simulink model "TEST_LIDAR"  (R2022b)
settings: Solver=FixedStepAuto  StartTime=0.0  StopTime=inf  FixedStep=1e-3  RelTol=1e-3  EnableMultiTasking=on
model workspace (MAT data in the model file):
  SL_ROS_VariableLengthArrays_MaxSizes : object (value not decoded)
values from neighbouring files (symbols this model uses):
  data = theClient.GetLastFrameOfData()    [FuncMotive.m]
undefined symbols (not defined in the file or in its folder): angular, carstamp, CIRCUIT, CLTF_DAMP, CLTF_FREQ, CLTF_GAIN, CONTROL, CONTROL_INI, DiscIntNeverNeededParam, INPUT, linear, MCP3201, MD25, MODEL, MODEL_INI, mpcstate, MPU60X0, MPU9250, MSG, NAV_MPC_CONTROL, OUTPUT, RCRX, SAMPLING_TIME, SYSID_INPUT, VL6180X
libraries: raspberrypiCommlib x160, simulink x89, raspberrypiNetworklib x22, ros2lib x14, dspsigattribs x14, embedlinuxBasiclib x12, ctrlSharedLib x2, mpclib x1, vrlib x1, sldrtlib x1
(part 13 of 19)

== matlab function TEST_LIDAR/CONTROL/STATE MACHINE UPDATE ==
  data: CONTROL_IN input Bus: CONTROL_Bus; CONTROL output Bus: CONTROL_Bus; MSG_IN input; MSG output Bus: MSG_Bus
function [CONTROL,MSG] = STATE_MACHINE(CONTROL_IN,MSG_IN)

%--------------------------------------------------------------
% COPY BUSES
%--------------------------------------------------------------
CONTROL = CONTROL_IN; 
MSG = MSG_IN;

%--------------------------------------------------------------
% TIMING
%--------------------------------------------------------------
% SAMPLING TIME
SAMPLING_TIME = CONTROL.PARAM.SAMPLING_TIME; % s
% 6-bit SAMPLING COUNTER
SAMPLING_COUNT = CONTROL.STATE.SAMPLING_COUNT;
SAMPLING_COUNT = SAMPLING_COUNT + uint8(1);
if SAMPLING_COUNT > uint8(63) 
    SAMPLING_COUNT = uint8(0);
end
CONTROL.STATE.SAMPLING_COUNT = SAMPLING_COUNT;
% TIMER
TIMER = CONTROL.STATE.TIMER;
% DELAY IN CONTROL ACTIVATION
CONTROL_ACT_DELAY = CONTROL.PARAM.CONTROL_ACT_DELAY;

%--------------------------------------------------------------
% SYSTEM OPERATION STATUS
%--------------------------------------------------------------
% / 0. BOOTING     / 1. SENSOR CALIBRATION / 2.  READY
% / 3. OPEN LOOP   / 4. ATTITUDE           / 5.  VELOCITY  
% / 6. NAVIGATION  / 7. WALL FOLLOWER      / 8.  NAVIGATION COMPETITION 
% / 9. WALL FOLLOWER COMPETITION           /10.  FORWARD VELOCITY COMPETITION
% /11. STOP        / 12. SELF-BALANCE      /13.  SBV CALIBRATION 
CURRENT_STATUS_SYS = CONTROL.STATE.CURRENT_STATUS_SYS;
NEXT_STATUS = CURRENT_STATUS_SYS;

%--------------------------------------------------------------
% PC OPERATION STATUS
%--------------------------------------------------------------
% / 0. CONTROL CONFIGURATION   / 1. WAITING FOR RPI SET UP  /
% / 2. MONITORIZATION / 3. STOP /
CURRENT_STATUS_PC = CONTROL.STATE.CURRENT_STATUS_PC;

%--------------------------------------------------------------
% CONTROL MODE
%--------------------------------------------------------------
% / 0. OPEN LOOP / 1. FORWARD VELOCITY AND YAW ANGLE / 
% / 2. FORWARD VELOCITY AND YAW RATE / 3. NAVIGATION / 
% / 4. WALL FOLLOWER / 5. WALL FOLLOWING COMPETITION /
% / 6. NAVIGATION COMPETITION / 7. FORWARD VELOCITY COMPETITION /
% / 8. SELF-BALANCE 
CONTROL_MODE = CONTROL.STATE.CONTROL_MODE;

%--------------------------------------------------------------
% CONTROL STATUS
%--------------------------------------------------------------
% / 0. INITIALIZATION  / 1. ESTIMATION  / 2. ACTIVE CONTROL
CONTROL_STATUS = CONTROL.STATE.CONTROL_STATUS;

%--------------------------------------------------------------
% MOTOR MODE
%--------------------------------------------------------------
% / 0. NOT ENABLED / 1. ENABLED 
MOTOR_MODE = CONTROL.STATE.MOTOR_MODE;

%--------------------------------------------------------------
% COMMUNICATIONS
%--------------------------------------------------------------
% COMMUNICATIONS MODE
% / 0. NOT ENABLED / 1. ENABLED / 2. BLACKBOX
COMM_MODE = CONTROL.STATE.COMM_MODE;
% UART MODE
% / 0. NOT ENABLED / 1. ENABLED
UART_MODE = CONTROL.STATE.UART_MODE;

%--------------------------------------------------------------
% INPUTS
%--------------------------------------------------------------
BUTTONS = CONTROL.STATE.BUTTONS;

%--------------------------------------------------------------
% PERSISTENT VARIABLES
%--------------------------------------------------------------
persistent initialize ACC_ERR MCS_EARTH_POS_OFFS MCS_EULER_ANG_OFFS ...
           NAV_EARTH_POS_OFFS NAV_EULER_ANG_OFFS IMU_PITCH_ANG_INI ...
           NUM_MSRT_LIDAR_2D TIMER_NAV
if isempty(initialize)
    ACC_ERR = 0;
    MCS_EARTH_POS_OFFS = zeros(3,1);
    MCS_EULER_ANG_OFFS = zeros(3,1);
    NAV_EARTH_POS_OFFS = zeros(3,1);
    NAV_EULER_ANG_OFFS = zeros(3,1);   
    IMU_PITCH_ANG_INI = 0;
    NUM_MSRT_LIDAR_2D = zeros(360,1);
    TIMER_NAV = 0;
    initialize = 1;
end

%--------------------------------------------------------------
% STATUS UPDATE
%--------------------------------------------------------------
switch CURRENT_STATUS_SYS
    
    %----------------------------------------------------------------------
    case 0 % BOOTING
    %----------------------------------------------------------------------
        % CONTROL STATUS: INITIALIZATION
        CONTROL_STATUS = uint8(0);     
        % MOTOR MODE: SHUTDOWN
        MOTOR_MODE = uint8(0);
        % LIDAR 2D
        if CONTROL.STATE.WALL_FOLLOWER_MODE
            CONTROL.STATE.LIDAR_2D_MODE = uint8(0);
        end
        % LEDs
        CONTROL.OUTPUT.LEDS = uint8([0 0 0]');
        % COMPETITION LIMITATION
        CONTROL.STATE.MAX_FORWARD_VEL_REACHED = uint8(0);
        % COMPETITION TIME AND ACCUMULATED ERROR
        CONTROL.STATE.COMP_TIME = 0;
        ACC_ERR = 0;
        % COMMUNICATIONS
        if COMM_MODE > 0
            BUFFER_RX = MSG.RX_BUFFER;
            NUM_MSG_RX = BUFFER_RX(1);
            if NUM_MSG_RX>0
                HEADER_RX = BUFFER_RX(1:2*NUM_MSG_RX+1);
                ID_RX = HEADER_RX(2:2:end);
                MSG.TX_ID = zeros(8,1,'uint8');
                if UART_MODE == 1
                    MSG.TX_ID(1:length(ID_RX)) = ID_RX(1:end)';
                else
                    MSG.TX_ID(1:length(ID_RX)) = [uint8(1) ID_RX(2:end)']';
                end
                if (BUTTONS(1) && (CURRENT_STATUS_PC == 1)) % BUTTON A
                    NEXT_STATUS = uint8(1); % SENSOR CALIBRATION
                    % TIMER RESET
                    TIMER = 0;
                end
            end
        else
            if BUTTONS(1) % BUTTON A
                NEXT_STATUS = uint8(1); % SENSOR CALIBRATION
                % TIMER RESET
                TIMER = 0;
            end
        end

    %----------------------------------------------------------------------
    case 1 % SENSOR CALIBRATION
    %----------------------------------------------------------------------
         % LIDAR 2D
        if CONTROL.STATE.WALL_FOLLOWER_MODE
            CONTROL.STATE.LIDAR_2D_MODE = uint8(1);
        end
        if TIMER >= 10
            if CONTROL.STATE.VEHICLE_MODE == 1 
                CONTROL.OUTPUT.LEDS = uint8([1 1 0]');
                if BUTTONS(1) % BUTTON A
                    NEXT_STATUS = uint8(13); % SVF CALIBRATION
                    % TIMER RESET
                    TIMER = 0;
                else
                    NEXT_STATUS = uint8(1); % SENSOR CALIBRATION
                end
            else
                NEXT_STATUS = uint8(2); % READY
            end
            % MOTION CAPTURE SYSTEM OFFSET
            CONTROL.PARAM.MCS_EARTH_POS_OFFS = MCS_EARTH_POS_OFFS;  
            CONTROL.PARAM.MCS_EULER_ANG_OFFS = MCS_EULER_ANG_OFFS; 
            % NAVIGATION SYSTEM OFFSET
            CONTROL.PARAM.NAV_EARTH_POS_OFFS = NAV_EARTH_POS_OFFS;
            CONTROL.PARAM.NAV_EULER_ANG_OFFS = NAV_EULER_ANG_OFFS;
        else
            % UPDATE TIMER
            TIMER = TIMER + SAMPLING_TIME;
            % LEDs
            CONTROL.OUTPUT.LEDS = uint8([0 0 1]');
            % MOTION CAPTURE SYSTEM CALIBRATION
            if CONTROL.STATE.MCS_MODE==1 || CONTROL.STATE.NAV_MODE==1
                ALFA_CALIB = CONTROL.PARAM.MCS_ALFA_CALIB;
                MCS_EARTH_POS_OFFS = ALFA_CALIB*MCS_EARTH_POS_OFFS + ...
                    (1-ALFA_CALIB)*CONTROL.INPUT.MCS_EARTH_POS;
                MCS_EULER_ANG_OFFS = ALFA_CALIB*MCS_EULER_ANG_OFFS + ...
                    (1-ALFA_CALIB)*CONTROL.INPUT.MCS_EULER_ANG;
            end            
            if CONTROL.STATE.NAV_MODE==3
                ALFA_CALIB = CONTROL.PARAM.NAV_ALFA_CALIB;
                NAV_EARTH_POS_OFFS = ALFA_CALIB*NAV_EARTH_POS_OFFS + ...
                    (1-ALFA_CALIB)*CONTROL.INPUT.NAV_EARTH_POS;
                NAV_EULER_ANG_OFFS = ALFA_CALIB*NAV_EULER_ANG_OFFS + ...
                    (1-ALFA_CALIB)*CONTROL.INPUT.NAV_EULER_ANG;
            end  
            if CONTROL.STATE.NAV_MODE==2
                for nn = 1:size(CONTROL.INPUT.LIDAR_2D,1)
                    if CONTROL.INPUT.LIDAR_2D(nn,2)>0
                        CONTROL.PARAM.LIDAR_2D_MAP(nn) = ...
                            (CONTROL.PARAM.LIDAR_2D_MAP(nn)*NUM_MSRT_LIDAR_2D(nn) + ...
                            CONTROL.INPUT.LIDAR_2D(nn,2))/(NUM_MSRT_LIDAR_2D(nn)+1);
                        NUM_MSRT_LIDAR_2D(nn) = NUM_MSRT_LIDAR_2D(nn) + 1;
                   end
                end
            end
        end
        % CONTROL STATUS: INITIALIZATION
        CONTROL_STATUS = uint8(0);     
        % MOTOR MODE: NOT ENABLED
        MOTOR_MODE = uint8(0); 
        % COMMUNICATIONS
        if (COMM_MODE >= 1) && (UART_MODE == 1)
            MSG.TX_ID = uint8([139 140 141 142 143 144 0 0]');
        elseif (COMM_MODE >= 1) && (UART_MODE == 0)
            MSG.TX_ID = uint8([1 139 140 141 142 143 144 0]');
        else
            MSG.TX_ID = uint8([0 0 0 0 0 0 0 0]');
        end

    %----------------------------------------------------------------------
    case 2 % READY
    %----------------------------------------------------------------------
        if BUTTONS(1) % BUTTON A
            if CONTROL_MODE == 0 % OPEN LOOP
                NEXT_STATUS = uint8(3); 
            elseif CONTROL_MODE == 1 % FORWARD VELOCITY AND YAW ANGLE
                NEXT_STATUS = uint8(4); 
            elseif CONTROL_MODE == 2 % FORWARD VELOCITY AND YAW RATE
                NEXT_STATUS = uint8(5); 
            elseif CONTROL_MODE == 3 % NAVIGATION
                NEXT_STATUS = uint8(6); 
            elseif CONTROL_MODE == 4 % WALL FOLLOWER
                NEXT_STATUS = uint8(7); 
            elseif CONTROL_MODE == 5 % WALL-FOLLOWER COMPETITION
                NEXT_STATUS = uint8(8); 
            elseif CONTROL_MODE == 6 % NAVIGATION COMPETITION
                NEXT_STATUS = uint8(9); 
            elseif CONTROL_MODE == 7 % FORWARD VELOCITY COMPETITION
                NEXT_STATUS = uint8(10);   
            elseif CONTROL_MODE == 8 % SELF-BALANCE
                NEXT_STATUS = uint8(12); 
            else
                NEXT_STATUS = uint8(11);
            end            
        end  
        % CONTROL STATUS: INITIALIZATION
        CONTROL_STATUS = uint8(0);              
        % MOTOR MODE: NOT ENABLED
        MOTOR_MODE = uint8(0); 
        % EKF MODE: NOT ENABLED
        CONTROL.EKF_IMU.ESTIMATION_MODE = uint8(0);
        CONTROL.EKF_WFL.ESTIMATION_MODE = uint8(0);
        % LEDs
        CONTROL.OUTPUT.LEDS = uint8([0 1 0]');
        % TARGETS
        CONTROL.TARGET.MOTOR_VOLT_CD_REF = zeros(2,1);
        CONTROL.TARGET.YAW_ANG_REF = 0;
        CONTROL.TARGET.FORWARD_VEL_REF = 0;
        CONTROL.TARGET.YAW_RATE_REF = 0;
        CONTROL.TARGET.WALL_DIST_REF = 0;
        % COMMUNICATIONS            
        if (COMM_MODE >= 1) && (UART_MODE == 1)
            MSG.TX_ID = uint8([139 140 141 142 143 144 0 0]');
        elseif (COMM_MODE >= 1) && (UART_MODE == 0)
            MSG.TX_ID = uint8([1 139 140 141 142 143 144 0]');
        else
            MSG.TX_ID = uint8([0 0 0 0 0 0 0 0]');
        end
        
    %----------------------------------------------------------------------
    case 3 % OPEN LOOP
    %----------------------------------------------------------------------
        if TIMER >= CONTROL_ACT_DELAY % Delay in control activation
            NEXT_STATUS = uint8(3);
            % CONTROL STATUS: ACTIVE CONTROL
            CONTROL_STATUS = uint8(2);
            % MOTOR MODE: ENABLED
            MOTOR_MODE = uint8(1);                       
           % LEDs
            CONTROL.OUTPUT.LEDS = uint8([0 0 0]');
            % TARGETS
            CONTROL.TARGET.MOTOR_VOLT_CD_REF = ...
                CONTROL.TARGET.MOTOR_VOLT_CD_REF_LC.*(CONTROL.STATE.MV_TARGET_SOURCE==0) + ...
                CONTROL.TARGET.MOTOR_VOLT_CD_REF_PC.*(CONTROL.STATE.MV_TARGET_SOURCE==1) + ...
                CONTROL.TARGET.MOTOR_VOLT_CD_REF_RC.*(CONTROL.STATE.MV_TARGET_SOURCE>=2);
            % BUTTON B
            if BUTTONS(2) == 1
                NEXT_STATUS = uint8(11); % STOP
                % TIMER_1 RESET
                TIMER = 0;                
            end
        else
            % UPDATE TIMER
            TIMER = TIMER + SAMPLING_TIME;
            % CONTROL STATUS: INITIALIZATION
            CONTROL_STATUS = uint8(0);
            % MOTOR MODE: NOT ENABLED
            MOTOR_MODE = uint8(0);
        end
        % COMMUNICATIONS
        if (COMM_MODE >= 1) && (UART_MODE == 1)
            MSG.TX_ID = uint8([139 140 141 142 143 144 0 0]');
        elseif (COMM_MODE >= 1) && (UART_MODE == 0)
            MSG.TX_ID = uint8([1 139 140 141 142 143 144 0]');
        else
            MSG.TX_ID = uint8([0 0 0 0 0 0 0 0]');
        end

    %----------------------------------------------------------------------
    case 4 % FORWARD VELOCITY AND YAW ANGLE
    %----------------------------------------------------------------------
        if TIMER >= CONTROL_ACT_DELAY % Delay in control activation
            NEXT_STATUS = uint8(4);
            % CONTROL STATUS: ACTIVE CONTROL
            CONTROL_STATUS = uint8(2);
            % MOTOR MODE: ENABLED
            MOTOR_MODE = uint8(1);                      
            % LEDs
            CONTROL.OUTPUT.LEDS = uint8([0 0 0]');
            % TARGETS
            CONTROL.TARGET.FORWARD_VEL_REF = ...
                CONTROL.TARGET.FORWARD_VEL_REF_LC.*(CONTROL.STATE.FV_TARGET_SOURCE==0) + ...
                CONTROL.TARGET.FORWARD_VEL_REF_PC.*(CONTROL.STATE.FV_TARGET_SOURCE==1) + ...
                CONTROL.TARGET.FORWARD_VEL_REF_RC.*(CONTROL.STATE.FV_TARGET_SOURCE>=2);
            CONTROL.TARGET.YAW_ANG_REF = ...
                CONTROL.TARGET.YAW_ANG_REF_LC.*(CONTROL.STATE.YA_TARGET_SOURCE==0) + ...
                CONTROL.TARGET.YAW_ANG_REF_PC.*(CONTROL.STATE.YA_TARGET_SOURCE==1) + ...
                CONTROL.TARGET.YAW_ANG_REF_RC.*(CONTROL.STATE.YA_TARGET_SOURCE>=2);
            % BUTTON B
            if BUTTONS(2) == 1
                NEXT_STATUS = uint8(11); % STOP
                % TIMER RESET
                TIMER = 0;                
            end
        else      
            % UPDATE TIMER
            TIMER = TIMER + SAMPLING_TIME;
            % CONTROL STATUS: INITIALIZATION
            CONTROL_STATUS = uint8(0);
            % MOTOR MODE: NOT ENABLED
            MOTOR_MODE = uint8(0);
        end
        % COMMUNICATIONS
        if (COMM_MODE >= 1) && (UART_MODE == 1)
            MSG.TX_ID = uint8([139 140 141 142 143 144 0 0]');
        elseif (COMM_MODE >= 1) && (UART_MODE == 0)
            MSG.TX_ID = uint8([1 139 140 141 142 143 144 0]');
        else
            MSG.TX_ID = uint8([0 0 0 0 0 0 0 0]');
        end

    %----------------------------------------------------------------------
    case 5 % FORWARD VELOCITY AND YAW RATE
    %----------------------------------------------------------------------
        if TIMER >= CONTROL_ACT_DELAY % Delay in control activation
            NEXT_STATUS = uint8(5);
            % CONTROL STATUS: ACTIVE CONTROL
            CONTROL_STATUS = uint8(2);
            % MOTOR MODE: ENABLED
            MOTOR_MODE = uint8(1);            
            % LEDs
            CONTROL.OUTPUT.LEDS = uint8([0 0 0]');
            % TARGETS
            CONTROL.TARGET.FORWARD_VEL_REF = ...
                CONTROL.TARGET.FORWARD_VEL_REF_LC.*(CONTROL.STATE.FV_TARGET_SOURCE==0) + ...
                CONTROL.TARGET.FORWARD_VEL_REF_PC.*(CONTROL.STATE.FV_TARGET_SOURCE==1) + ...
                CONTROL.TARGET.FORWARD_VEL_REF_RC.*(CONTROL.STATE.FV_TARGET_SOURCE>=2);
            CONTROL.TARGET.YAW_RATE_REF = ...
                CONTROL.TARGET.YAW_RATE_REF_LC.*(CONTROL.STATE.YR_TARGET_SOURCE==0) + ...
                CONTROL.TARGET.YAW_RATE_REF_PC.*(CONTROL.STATE.YR_TARGET_SOURCE==1) + ...
                CONTROL.TARGET.YAW_RATE_REF_RC.*(CONTROL.STATE.YR_TARGET_SOURCE>=2);
            % BUTTON B
            if BUTTONS(2) == 1
                NEXT_STATUS = uint8(11); % STOP
                % TIMER RESET
                TIMER = 0;                
            end
        else      
            % UPDATE TIMER
            TIMER = TIMER + SAMPLING_TIME;
            % CONTROL STATUS: INITIALIZATION
            CONTROL_STATUS = uint8(0);
            % MOTOR MODE: NOT ENABLED
            MOTOR_MODE = uint8(0);
        end
         % COMMUNICATIONS
        if (COMM_MODE >= 1) && (UART_MODE == 1)
            MSG.TX_ID = uint8([139 140 141 142 143 144 0 0]');
        elseif (COMM_MODE >= 1) && (UART_MODE == 0)
            MSG.TX_ID = uint8([1 139 140 141 142 143 144 0]');
        else
            MSG.TX_ID = uint8([0 0 0 0 0 0 0 0]');
        end

    %----------------------------------------------------------------------
    case 6 % NAVIGATION
    %----------------------------------------------------------------------
        if TIMER >= CONTROL_ACT_DELAY % Delay in control activation
            NEXT_STATUS = uint8(6);
            % CONTROL STATUS: ACTIVE CONTROL
            CONTROL_STATUS = uint8(2);
            % MOTOR MODE: ENABLED
            MOTOR_MODE = uint8(1);
            % BUTTON B
            if BUTTONS(2) == 1
                NEXT_STATUS = uint8(11); % STOP
                % TIMER RESET
                TIMER = 0;                
            end
            % LEDs
            CONTROL.OUTPUT.LEDS = uint8([0 0 0]');
            % TARGETS
            if CONTROL.STATE.NAV_TARGET_SOURCE==0 % LOCAL
                CONTROL.TARGET.NAV_REF = CONTROL.TARGET.NAV_REF_LC;
            elseif CONTROL.STATE.NAV_TARGET_SOURCE==1 % PC
                CONTROL.TARGET.NAV_REF = CONTROL.TARGET.NAV_REF_PC;
            elseif CONTROL.STATE.NAV_TARGET_SOURCE==2 || CONTROL.STATE.NAV_TARGET_SOURCE==3 % RC
                CONTROL.TARGET.NAV_REF = CONTROL.TARGET.NAV_REF_RC;
            elseif CONTROL.STATE.NAV_TARGET_SOURCE==4 % MISSION
                % Number of waypoints
                NUM_WAYPOINTS = CONTROL.PARAM.MISSION_NUM_WAYPOINTS;
                % Waypoint list
                WP_LIST = CONTROL.PARAM.MISSION_WAYPOINTS(1:NUM_WAYPOINTS,:);
                % Next waypoint
                NEXT_WP = CONTROL.PARAM.MISSION_COUNT;
                % Tolerances
                WP_RADIUS = CONTROL.PARAM.MISSION_WP_RADIUS;
                % References
                CONTROL.TARGET.NAV_REF = WP_LIST(NEXT_WP,2:3)';
                % POSITION UPDATE
                % Current position and yaw angle
                NAV_MO = CONTROL.INPUT.NAV_MO;
                % Check waypoint
                POS_DIST = sqrt(sum((CONTROL.TARGET.NAV_REF - NAV_MO).^2));
                % Increase waypoint
                if POS_DIST<WP_RADIUS
                    if WP_LIST(NEXT_WP,1)>TIMER_NAV
                        TIMER_NAV = TIMER_NAV + SAMPLING_TIME;
                    else
                        TIMER_NAV = 0;
                        NEXT_WP = NEXT_WP + uint8(1);
                    end
                end
                if NEXT_WP>size(WP_LIST,1)
                    NEXT_WP = uint8(size(WP_LIST,1));
                end
                % CONTROL BUS UPDATE FOR COMPETITION
                CONTROL.PARAM.MISSION_COUNT = NEXT_WP;
            else
                % NEXT STATUS: READY
                NEXT_STATUS = uint8(2);
                % MOTOR MODE: SHUT DOWN
                MOTOR_MODE = uint8(0);
            end
            CONTROL.TARGET.POS_XY_REF = CONTROL.TARGET.NAV_REF;
            % BUTTON B
            if BUTTONS(2) == 1
                NEXT_STATUS = uint8(11); % STOP
                % TIMER RESET
                TIMER = 0;
            end
        else
            % UPDATE TIMER
            TIMER = TIMER + SAMPLING_TIME;
            % CONTROL STATUS: INITIALIZATION
            CONTROL_STATUS = uint8(0);
            % MOTOR MODE: NOT ENABLED
            MOTOR_MODE = uint8(0);
        end
        % COMMUNICATIONS
        if (COMM_MODE >= 1) && (UART_MODE == 1)
            MSG.TX_ID = uint8([139 140 141 142 143 144 0 0]');
        elseif (COMM_MODE >= 1) && (UART_MODE == 0)
            MSG.TX_ID = uint8([1 139 140 141 142 143 144 0]');
        else
            MSG.TX_ID = uint8([0 0 0 0 0 0 0 0]');
        end
        
    %----------------------------------------------------------------------
    case 7 % WALL FOLLOWER
    %----------------------------------------------------------------------
        if TIMER >= CONTROL_ACT_DELAY % Delay in control activation
            NEXT_STATUS = uint8(7);
            % CONTROL STATUS: ACTIVE CONTROL
            CONTROL_STATUS = uint8(2);
            % MOTOR MODE: ENABLED
            MOTOR_MODE = uint8(1); 
            % LIDAR 2D
            if CONTROL.STATE.WALL_FOLLOWER_MODE
                CONTROL.STATE.LIDAR_2D_MODE = uint8(1);
            end
            % LEDs
            CONTROL.OUTPUT.LEDS = uint8([0 0 0]');
            % TARGETS
            CONTROL.TARGET.FORWARD_VEL_REF = ...
                CONTROL.TARGET.FORWARD_VEL_REF_LC.*(CONTROL.STATE.FV_TARGET_SOURCE==0) + ...
                CONTROL.TARGET.FORWARD_VEL_REF_PC.*(CONTROL.STATE.FV_TARGET_SOURCE==1) + ...
                CONTROL.TARGET.FORWARD_VEL_REF_RC.*(CONTROL.STATE.FV_TARGET_SOURCE>=2);
            CONTROL.TARGET.WALL_DIST_REF = ...
                CONTROL.TARGET.WALL_DIST_REF_LC.*(CONTROL.STATE.WD_TARGET_SOURCE==0) + ...
                CONTROL.TARGET.WALL_DIST_REF_PC.*(CONTROL.STATE.WD_TARGET_SOURCE==1) + ...
                CONTROL.TARGET.WALL_DIST_REF_RC.*(CONTROL.STATE.WD_TARGET_SOURCE>=2);
            % BUTTON B
            if BUTTONS(2) == 1
                NEXT_STATUS = uint8(11); % STOP
                % TIMER RESET
                TIMER = 0;                
            end
        else      
            % UPDATE TIMER
            TIMER = TIMER + SAMPLING_TIME;
            % CONTROL STATUS: INITIALIZATION
            CONTROL_STATUS = uint8(0);
            % MOTOR MODE: NOT ENABLED
            MOTOR_MODE = uint8(0);
        end        
        % COMMUNICATIONS
        if (COMM_MODE >= 1) && (UART_MODE == 1)
            MSG.TX_ID = uint8([139 140 141 142 143 144 0 0]');
        elseif (COMM_MODE >= 1) && (UART_MODE == 0)
            MSG.TX_ID = uint8([1 139 140 141 142 143 144 0]');
        else
            MSG.TX_ID = uint8([0 0 0 0 0 0 0 0]');
        end

    %----------------------------------------------------------------------
    case 8 % WALL-FOLLOWER COMPETITION
    %----------------------------------------------------------------------
        if TIMER >= CONTROL_ACT_DELAY % Delay in control activation
            NEXT_STATUS = uint8(8);
            % CONTROL STATUS: ACTIVE CONTROL
            CONTROL_STATUS = uint8(2);
            % MOTOR MODE: ENABLED
            MOTOR_MODE = uint8(1);
            % LIDAR 2D
            if CONTROL.STATE.WALL_FOLLOWER_MODE
                CONTROL.STATE.LIDAR_2D_MODE = uint8(1);
            end            % LEDs
            CONTROL.OUTPUT.LEDS = uint8([0 0 0]');
            % TARGETS
            CONTROL.TARGET.FORWARD_VEL_REF = ...
                CONTROL.TARGET.FORWARD_VEL_REF_LC.*(CONTROL.STATE.FV_TARGET_SOURCE==0) + ...
                CONTROL.TARGET.FORWARD_VEL_REF_PC.*(CONTROL.STATE.FV_TARGET_SOURCE==1) + ...
                CONTROL.TARGET.FORWARD_VEL_REF_RC.*(CONTROL.STATE.FV_TARGET_SOURCE>=2);
            CONTROL.TARGET.WALL_DIST_REF = ...
                CONTROL.TARGET.WALL_DIST_REF_LC.*(CONTROL.STATE.WD_TARGET_SOURCE==0) + ...
                CONTROL.TARGET.WALL_DIST_REF_PC.*(CONTROL.STATE.WD_TARGET_SOURCE==1) + ...
                CONTROL.TARGET.WALL_DIST_REF_RC.*(CONTROL.STATE.WD_TARGET_SOURCE>=2);       
            % FORWARD VELOCITY LIMITATION
            if CONTROL.INPUT.FORWARD_VEL>0.5
                CONTROL.STATE.MAX_FORWARD_VEL_REACHED = uint8(1);
            end
            if CONTROL.STATE.MAX_FORWARD_VEL_REACHED
                CONTROL.TARGET.FORWARD_VEL_REF = 0;
            end
            % BUTTON B
            if BUTTONS(2) == 1
                NEXT_STATUS = uint8(11); % STOP
                % TIMER RESET
                TIMER = 0;                
            end
        else      
            % UPDATE TIMER
            TIMER = TIMER + SAMPLING_TIME;
            % CONTROL STATUS: INITIALIZATION
            CONTROL_STATUS = uint8(0);
            % MOTOR MODE: NOT ENABLED
            MOTOR_MODE = uint8(0);
        end
        % COMMUNICATIONS
        if (COMM_MODE >= 1) && (UART_MODE == 1)
            MSG.TX_ID = uint8([139 140 141 142 143 144 0 0]');
        elseif (COMM_MODE >= 1) && (UART_MODE == 0)
            MSG.TX_ID = uint8([1 139 140 141 142 143 144 0]');
        else
            MSG.TX_ID = uint8([0 0 0 0 0 0 0 0]');
        end

    %----------------------------------------------------------------------
    case 9 % NAVIGATION COMPETITION
    %----------------------------------------------------------------------
        if TIMER >= CONTROL_ACT_DELAY % Delay in control activation
            NEXT_STATUS = uint8(9);
            % CONTROL STATUS: ACTIVE CONTROL
            CONTROL_STATUS = uint8(2);
            % MOTOR MODE: ENABLED
            MOTOR_MODE = uint8(1);
            % BUTTON B
            if BUTTONS(2) == 1
                NEXT_STATUS = uint8(11); % STOP
                % TIMER RESET
                TIMER = 0;                
            end
            % LEDs
            CONTROL.OUTPUT.LEDS = uint8([0 0 0]');
            % POSITION UPDATE
            WP_XY = CONTROL.PARAM.MISSION_WAYPOINTS(1:CONTROL.PARAM.MISSION_NUM_WAYPOINTS,2:3)';
            WP_R = CONTROL.PARAM.MISSION_WP_RADIUS;
            NAV_MO = CONTROL.INPUT.NAV_MO;
            NEXT_WP = CONTROL.PARAM.MISSION_COUNT;
            POS_INC = (WP_XY(1,NEXT_WP) - NAV_MO(1)) + (WP_XY(2,NEXT_WP) - NAV_MO(2))*1i;
            POS_INC_MAG = abs(POS_INC);
            % COMPETITION TIME UPDATE
            COMP_START_TIME = CONTROL.STATE.COMP_START_TIME;
            COMP_TIME = CONTROL.STATE.COMP_TIME;
            if COMP_START_TIME>0 && POS_INC_MAG<WP_R && NEXT_WP==1
                CONTROL.STATE.COMP_STARTED = uint8(1);
            end
            if CONTROL.STATE.COMP_STARTED && CONTROL.STATE.COMP_FINISHED==0
                COMP_TIME = COMP_TIME + SAMPLING_TIME;
            else
                COMP_START_TIME = COMP_START_TIME + SAMPLING_TIME*(CONTROL.STATE.COMP_STARTED==0);
            end
            if POS_INC_MAG<WP_R && CONTROL.STATE.COMP_STARTED
                 NEXT_WP = NEXT_WP + uint8(1);
            end
            if NEXT_WP>size(WP_XY,2)
                NEXT_WP = uint8(size(WP_XY,2));
                CONTROL.STATE.COMP_FINISHED = uint8(1);
                CONTROL.TARGET.NAV_REF(1) = 0;               
            end
            % CONTROL BUS UPDATE FOR COMPETITION   
            CONTROL.TARGET.NAV_REF = WP_XY(:,NEXT_WP);
            CONTROL.TARGET.POS_XY_REF = CONTROL.TARGET.NAV_REF;
            CONTROL.PARAM.MISSION_COUNT = NEXT_WP;
            CONTROL.STATE.COMP_START_TIME = COMP_START_TIME;
            CONTROL.STATE.COMP_TIME = COMP_TIME;
        else      
            % UPDATE TIMER
            TIMER = TIMER + SAMPLING_TIME;
            % CONTROL STATUS: INITIALIZATION
            CONTROL_STATUS = uint8(0);
            % MOTOR MODE: NOT ENABLED
            MOTOR_MODE = uint8(0);
        end
        % COMMUNICATIONS
        if (COMM_MODE >= 1) && (UART_MODE == 1)
            MSG.TX_ID = uint8([139 140 141 142 143 144 0 0]');
        elseif (COMM_MODE >= 1) && (UART_MODE == 0)
            MSG.TX_ID = uint8([1 139 140 141 142 143 144 0]');
        else
            MSG.TX_ID = uint8([0 0 0 0 0 0 0 0]');
        end
        
    %----------------------------------------------------------------------
    case 10 % FORWARD VELOCITY COMPETITION
    %----------------------------------------------------------------------
        if TIMER >= CONTROL_ACT_DELAY % Delay in control activation
            NEXT_STATUS = uint8(10);
            % CONTROL STATUS: ACTIVE CONTROL
            CONTROL_STATUS = uint8(2);
            % MOTOR MODE: ENABLED
            MOTOR_MODE = uint8(1);                      
            % LEDs
            CONTROL.OUTPUT.LEDS = uint8([0 0 0]');
            % TARGETS
            CONTROL.TARGET.FORWARD_VEL_REF = CONTROL.TARGET.FORWARD_VEL_REF_LC;
            CONTROL.TARGET.YAW_RATE_REF = CONTROL.TARGET.YAW_RATE_REF_LC;
            % COMPETITION TIME
            COMP_TIME = CONTROL.STATE.COMP_TIME;
            COMP_TIME = COMP_TIME + SAMPLING_TIME;
            % IAE COMPUTATION
            if COMP_TIME >= 5
                ACC_ERR = ACC_ERR +  abs(CONTROL.TARGET.FORWARD_VEL_REF - CONTROL.INPUT.FORWARD_VEL);    
            end
            % BUTTON B
            if BUTTONS(2) == 1 || COMP_TIME >= 20
                NEXT_STATUS = uint8(11); % STOP
                % TIMER RESET
                TIMER = 0;                
            end
            % CONTROL BUS UPDATE FOR COMPETITION   
            CONTROL.STATE.COMP_TIME = COMP_TIME;
            CONTROL.STATE.COMP_IAE = ACC_ERR/(COMP_TIME-5)*SAMPLING_TIME*300000;
        else      
            % UPDATE TIMER
            TIMER = TIMER + SAMPLING_TIME;
            % CONTROL STATUS: INITIALIZATION
            CONTROL_STATUS = uint8(0);
            % MOTOR MODE: NOT ENABLED
            MOTOR_MODE = uint8(0);
        end
        % COMMUNICATIONS
        if (COMM_MODE >= 1) && (UART_MODE == 1)
            MSG.TX_ID = uint8([139 140 141 142 143 144 0 0]');
        elseif (COMM_MODE >= 1) && (UART_MODE == 0)
            MSG.TX_ID = uint8([1 139 140 141 142 143 144 0]');
        else
            MSG.TX_ID = uint8([0 0 0 0 0 0 0 0]');
        end

    %----------------------------------------------------------------------
    case 12 % SELF-BALANCE
    %----------------------------------------------------------------------
        if TIMER >= CONTROL_ACT_DELAY % Delay in control activation
            NEXT_STATUS = uint8(12);
            % CONTROL STATUS: ACTIVE CONTROL
            CONTROL_STATUS = uint8(2);
            % MOTOR MODE: ENABLED
            MOTOR_MODE = uint8(1);                      
            % LEDs
            CONTROL.OUTPUT.LEDS = uint8([0 0 0]');
            % BUTTON B
            if BUTTONS(2) == 1
                NEXT_STATUS = uint8(11); % STOP
                % TIMER RESET
                TIMER = 0;                
            end
        else      
            % UPDATE TIMER
            TIMER = TIMER + SAMPLING_TIME;
            % CONTROL STATUS: INITIALIZATION
            CONTROL_STATUS = uint8(0);
            % MOTOR MODE: NOT ENABLED
            MOTOR_MODE = uint8(0);
        end
        % COMMUNICATIONS
        if (COMM_MODE >= 1) && (UART_MODE == 1)
            MSG.TX_ID = uint8([139 140 141 142 143 144 0 0]');
        elseif (COMM_MODE >= 1) && (UART_MODE == 0)
            MSG.TX_ID = uint8([1 139 140 141 142 143 144 0]');
        else
            MSG.TX_ID = uint8([0 0 0 0 0 0 0 0]');
        end

    %----------------------------------------------------------------------
    case 13 % SELF-BALANCING VEHICLE CALIBRATION
    %----------------------------------------------------------------------
        if TIMER >= 2 && abs(IMU_PITCH_ANG_INI - CONTROL.PARAM.IMU_PITCH_OFFSET)<=CONTROL.PARAM.PA_INITIAL_VALUE
            NEXT_STATUS = uint8(2); % READY
            % TIMER RESET
            TIMER = 0;
            % UPDATE INITIAL PITCH ANGLE
            CONTROL.INPUT.IMU_PITCH_ANG_INI = IMU_PITCH_ANG_INI - CONTROL.PARAM.IMU_PITCH_OFFSET;            
        else
            % UPDATE TIMER
            TIMER = TIMER + SAMPLING_TIME;
            % IMU IN Z-AXIS CALIBRATION (PITCH ANGLE)
            ALFA_CALIB = 0.95;
            IMU_PITCH_ANG_INI = ALFA_CALIB*IMU_PITCH_ANG_INI + ...
                (1-ALFA_CALIB)*atan2(CONTROL.INPUT.IMU_ACCEL_MEAN_FILT(3),CONTROL.INPUT.IMU_ACCEL_MEAN_FILT(1));
        end
        % LEDs
        CONTROL.OUTPUT.LEDS = uint8([0 0 1]');
        % CONTROL STATUS: INITIALIZATION
        CONTROL_STATUS = uint8(0);     
        % MOTOR MODE: NOT ENABLED
        MOTOR_MODE = uint8(0); 
        % COMMUNICATIONS
        if (COMM_MODE >= 1) && (UART_MODE == 1)
            MSG.TX_ID = uint8([139 140 141 142 143 144 0 0]');
        elseif (COMM_MODE >= 1) && (UART_MODE == 0)
            MSG.TX_ID = uint8([1 139 140 141 142 143 144 0]');
        else
            MSG.TX_ID = uint8([0 0 0 0 0 0 0 0]');
        end
        
    %----------------------------------------------------------------------
    case 11 % STOP
    %----------------------------------------------------------------------
        % CONTROL STATUS: INITIALIZATION
        CONTROL_STATUS = uint8(0);     
        % MOTOR MODE: NOT ENABLED
        MOTOR_MODE = uint8(0);                        
        % LIDAR 2D
        if CONTROL.STATE.WALL_FOLLOWER_MODE
            CONTROL.STATE.LIDAR_2D_MODE = uint8(0);
        end
        % COMPETITION LIMITATION
        CONTROL.STATE.MAX_FORWARD_VEL_REACHED = uint8(0);
        % LEDs: RED 
        CONTROL.OUTPUT.LEDS = uint8([1 0 0]');
        % BUTTON C
        if BUTTONS(3) == 1
            NEXT_STATUS = uint8(0); % BOOTING
        end
        % COMMUNICATIONS
        if (COMM_MODE >= 1) && (UART_MODE == 1)
            MSG.TX_ID = uint8([139 140 141 142 143 144 0 0]');
        elseif (COMM_MODE >= 1) && (UART_MODE == 0)
            MSG.TX_ID = uint8([1 139 140 141 142 143 144 0]');
        else
            MSG.TX_ID = uint8([0 0 0 0 0 0 0 0]');
        end
end

%--------------------------------------------------------------
% CONTROL BUS UPDATE
%--------------------------------------------------------------
CONTROL.STATE.CURRENT_STATUS_SYS = NEXT_STATUS;
CONTROL.STATE.PREVIOUS_STATUS = CURRENT_STATUS_SYS;
CONTROL.STATE.CONTROL_STATUS = CONTROL_STATUS;
CONTROL.STATE.MOTOR_MODE = MOTOR_MODE;
CONTROL.STATE.TIMER = TIMER;
CONTROL.PARAM.MCS_EARTH_POS_OFFS = MCS_EARTH_POS_OFFS;
CONTROL.PARAM.MCS_EULER_ANG_OFFS = MCS_EULER_ANG_OFFS;
CONTROL.PARAM.NAV_EARTH_POS_OFFS = NAV_EARTH_POS_OFFS;
CONTROL.PARAM.NAV_EULER_ANG_OFFS = NAV_EULER_ANG_OFFS;

== matlab function TEST_LIDAR/CONTROL/LOCAL TARGETS/YAW ANGLE TARGET/ PULSE GENERATION ==
  data: CONTROL input Bus: CONTROL_Bus; YAW_ANG_REF output
function YAW_ANG_REF = PULSE_GEN(CONTROL)
    
persistent TIMER initialize
if isempty(initialize)
    TIMER = 0;
    initialize = 1;
end

% SAMPLING TIME
SAMPLING_TIME = CONTROL.PARAM.SAMPLING_TIME; % s

%% OPERATION MODE
% / 0. BOOTING   / 1. SENSOR CALIBRATION / 2. READY
% / 3. OPEN LOOP / 4. ATTITUDE / 5. VELOCITY / 6. NAVIGATION / 
% / 7. WALL FOLLOWER / 8. WALL-FOLLOWER COMPETITION / 
% / 9. NAVIGATION COMPETITION / 10. STOP
CURRENT_STATUS = CONTROL.STATE.CURRENT_STATUS_SYS;
PREVIOUS_STATUS = CONTROL.STATE.PREVIOUS_STATUS;

if (CURRENT_STATUS == 4) && (PREVIOUS_STATUS == 4)   
    if TIMER > 3
        YAW_ANG_REF = 0;
    elseif TIMER < 0.5
        YAW_ANG_REF = 0;
        TIMER = TIMER + SAMPLING_TIME;
    else % 0.5 <= TIMER <= 3
        YAW_ANG_REF = 60*pi/180;
        TIMER = TIMER + SAMPLING_TIME;
    end
else
    YAW_ANG_REF = 0;
    TIMER = 0;
end

== matlab function TEST_LIDAR/HARDWARE/ACTUATORS/MD25_I2C/READ MOTOR ENCODER/READ_ENCODER ==
  data: CONTROL_IN input Bus: CONTROL_Bus; MOTOR_ENC_BYTES input; CONTROL output Bus: CONTROL_Bus
function CONTROL = READ_ENCODER(CONTROL_IN,MOTOR_ENC_BYTES)

%--------------------------------------------------------------
% UPDATE BUS
%--------------------------------------------------------------
CONTROL = CONTROL_IN;

%--------------------------------------------------------------
% STATE
%--------------------------------------------------------------
persistent initialize left_enc_prv right_enc_prv inc_com_ang_prv ...
           inc_dif_ang_prv inc2_com_ang_prv inc2_dif_ang_prv dif_ang ...
           dif_ang_offs left_enc_offs right_enc_offs

if isempty(initialize)
    left_enc_prv = zeros(2,1);
    right_enc_prv = zeros(2,1);
    left_enc_offs = 0;
    right_enc_offs = 0;
    inc_com_ang_prv = zeros(5,1);
    inc_dif_ang_prv = zeros(5,1);
    inc2_com_ang_prv = zeros(5,1);
    inc2_dif_ang_prv = zeros(5,1);
    dif_ang = 0;
    dif_ang_offs = 0;        
    initialize = 1;
end

%--------------------------------------------------------------
% PARAMETERS
%--------------------------------------------------------------
% Wheel gear ratio
WHEEL_GEAR_RATIO = CONTROL.PARAM.WHEEL_GEAR_RATIO;
% Motor gear ratio
MOTOR_GEAR_RATIO = CONTROL.PARAM.MOTOR_GEAR_RATIO;
% Encoder resolution: number of pulses / revolution of main shaft
MOTOR_ENC_RES = CONTROL.PARAM.MOTOR_ENC_RES; 

%--------------------------------------------------------------
% ENCODER READOUT
%--------------------------------------------------------------
right_enc = -double(typecast(MOTOR_ENC_BYTES([4 3 2 1],1),'int32'));
left_enc = -double(typecast(MOTOR_ENC_BYTES([8 7 6 5],1),'int32')); 
inc_right_enc = right_enc - right_enc_prv(1);
inc_left_enc = left_enc - left_enc_prv(1);
inc2_right_enc = right_enc - 2*right_enc_prv(1) + right_enc_prv(2);
inc2_left_enc = left_enc - 2*left_enc_prv(1) + left_enc_prv(2);
inc_right_ang = 360/MOTOR_ENC_RES/MOTOR_GEAR_RATIO/WHEEL_GEAR_RATIO*inc_right_enc;
inc_left_ang = 360/MOTOR_ENC_RES/MOTOR_GEAR_RATIO/WHEEL_GEAR_RATIO*inc_left_enc;
inc2_right_ang = 360/MOTOR_ENC_RES/MOTOR_GEAR_RATIO/WHEEL_GEAR_RATIO*inc2_right_enc;
inc2_left_ang = 360/MOTOR_ENC_RES/MOTOR_GEAR_RATIO/WHEEL_GEAR_RATIO*inc2_left_enc;
inc_com_ang = (inc_left_ang + inc_right_ang)/2;
inc_dif_ang = (inc_left_ang - inc_right_ang)/2;
inc2_com_ang = (inc2_left_ang + inc2_right_ang)/2;
inc2_dif_ang = (inc2_left_ang - inc2_right_ang)/2;
% Define first-order incremental encoder threshold 
THR_INC_ENC_DEG = 10; 
% Define second-order incremental encoder threshold 
THR_INC2_ENC_DEG = 1; 
% Check incremental limits
if (abs(inc_right_ang)>THR_INC_ENC_DEG)   || ...
   (abs(inc_left_ang)>THR_INC_ENC_DEG)    || ...
   (abs(inc2_right_ang)>THR_INC2_ENC_DEG) || ...
   (abs(inc2_left_ang)>THR_INC2_ENC_DEG)
    inc2_com_ang = mean(inc2_com_ang_prv);
    inc2_dif_ang = mean(inc2_dif_ang_prv);
    inc_com_ang = mean(inc_com_ang_prv) + inc2_com_ang;
    inc_dif_ang = mean(inc_dif_ang_prv) + inc2_dif_ang;
end
% Update differential angles
dif_ang = dif_ang + inc_dif_ang;
% Update previous values
left_enc_prv(2) = left_enc_prv(1);
right_enc_prv(2) = right_enc_prv(1);
left_enc_prv(1) = left_enc;
right_enc_prv(1) = right_enc;
inc_com_ang_prv = [inc_com_ang ; inc_com_ang_prv(1:end-1)];
inc_dif_ang_prv = [inc_dif_ang ; inc_dif_ang_prv(1:end-1)];
inc2_com_ang_prv = [inc2_com_ang ; inc2_com_ang_prv(1:end-1)];
inc2_dif_ang_prv = [inc2_dif_ang ; inc2_dif_ang_prv(1:end-1)];

%--------------------------------------------------------------
% CALIBRATION 
%--------------------------------------------------------------
ALFA_CALIB = 0.99;
if CONTROL.STATE.CURRENT_STATUS_SYS == 1  % CALIBRATION ENABLED
    dif_ang_offs  = ALFA_CALIB*dif_ang_offs  + (1-ALFA_CALIB)*dif_ang;
    left_enc_offs = ALFA_CALIB*left_enc_offs  + (1-ALFA_CALIB)*left_enc;
    right_enc_offs = ALFA_CALIB*right_enc_offs  + (1-ALFA_CALIB)*right_enc;
elseif CONTROL.STATE.CURRENT_STATUS_SYS == 0
    return
else
end 

%--------------------------------------------------------------
% ENCODER ANGLES
%--------------------------------------------------------------
CONTROL.INPUT.ENC_INC2_COM_ANG = inc2_com_ang;
CONTROL.INPUT.ENC_INC2_DIF_ANG = inc2_dif_ang;
CONTROL.INPUT.ENC_INC_COM_ANG = inc_com_ang;
CONTROL.INPUT.ENC_INC_DIF_ANG = inc_dif_ang;
CONTROL.INPUT.ENC_DIF_ANG = dif_ang-dif_ang_offs;
CONTROL.INPUT.ENC_MOTOR_ANG = 2*pi/MOTOR_ENC_RES/MOTOR_GEAR_RATIO/WHEEL_GEAR_RATIO*[left_enc-left_enc_offs right_enc-right_enc_offs]';

return

== matlab function TEST_LIDAR/CONTROL/SYSTEM IDENTIFICATION/Second-order equation1 ==
  data: b input; r1 output; c input; r2 output
function [r1,r2] = sol_2ord_eq(b,c)
r1 = (-b+sqrt(abs(b^2-4*c)))/2;
r2 = (-b-sqrt(abs(b^2-4*c)))/2;
return

== matlab function TEST_LIDAR/SIMULATION/CIRCUIT/CIRCUITO ==
  data: xi input; yi input; d output; theta input; param input; est_ant input; theta_circ output; d1 output; d2 output; rampa output; estado output
function [d,theta_circ,d1,d2,rampa,estado] = fcn(xi,yi,theta,param,est_ant)

%% Parametros
L=param(1); % Longitud tramo recto
Lr=param(2); % Longitud rampa
R=param(3);  % Radio de la curva
d_sens=param(4); % Distancia entre sensores

% Sensor delantero
xid=xi+d_sens/2*cos(theta);
yid=yi+d_sens/2*sin(theta);
% Sensor trasero
xit=xi-d_sens/2*cos(theta);
yit=yi-d_sens/2*sin(theta);
% Ecuacion de la recta normal
% y-yi = tan(theta-pi/2)*(x-xi)

%% Distancia del sensor delantero
% Corte con el tramo recto de la pared del circuito
% x=xi+(sign(yi)*R-yi)/tan(theta-pi/2)
x_1=[xid+(R-yid)/tan(theta-pi/2); xid+(-R-yid)/tan(theta-pi/2)];
y_1=[R; -R];
V1=(x_1-xid)+1j*(y_1-yid);
V2=d_sens/2*cos(theta)+1j*d_sens/2*sin(theta);
ang_1=angle(V2./V1)*180/pi;
[~,ind]=min(abs(ang_1-90));
x_1=x_1(ind);
y_1=y_1(ind);
% Corte con la curva del circuito
% (yi+tan(theta-pi/2)*(x-xi))^2 = R^2-(x-sign(xi)*L/2)^2
% yi^2+tan(theta-pi/2)^2*(x^2+xi^2-2*xi*x)+2*tan(theta-pi/2)*(x-xi)*yi = R^2-x^2-L^2/4+2*sign(xi)*L/2*x
% x = roots([tan(theta-pi/2)^2+1  -2*(xi*tan(theta-pi/2)^2+sign(xi)*L/2-tan(theta-pi/2)*yi)   yi^2+tan(theta-pi/2)^2*xi^2-R^2+L^2/4-2*tan(theta-pi/2)*xi*yi])
if abs(x_1)<=L/2
    xcd=x_1;
    ycd=y_1;
else
    x_2 = roots([tan(theta-pi/2)^2+1 ...
        -2*(xid*tan(theta-pi/2)^2+sign(xid)*L/2-tan(theta-pi/2)*yid) ...
        yid^2+tan(theta-pi/2)^2*xid^2-R^2+L^2/4-2*tan(theta-pi/2)*xid*yid]);
        [~,ind]=min(abs(x_2-xid));
    xcd=x_2(ind);
    aux=sqrt(abs(R^2-(xcd-sign(xid)*L/2)^2));
    y_2=[aux ; -aux];
    V1=[(xcd-xid)+1j*(y_2(1)-yid) ; (xcd-xid)+1j*(y_2(2)-yid)];
    V2=[d_sens/2*cos(theta)+1j*d_sens/2*sin(theta); d_sens/2*cos(theta)+1j*d_sens/2*sin(theta)];
    ang_2=angle(V2./V1)*180/pi;
    [~,ind]=min(abs(ang_2-90));
    ycd=y_2(ind);
end
d1=norm([xcd-xid ; ycd-yid]);

%% Distancia del sensor trasero
% Corte con el tramo recto de la pared del circuito
% x=xi+(sign(yi)*R-yi)/tan(theta-pi/2)
x_1=[xit+(R-yit)/tan(theta-pi/2); xit+(-R-yit)/tan(theta-pi/2)];
y_1=[R; -R];
V1=(x_1-xit)+1j*(y_1-yit);
V2=d_sens/2*cos(theta)+1j*d_sens/2*sin(theta);
ang_1=angle(V2./V1)*180/pi;
[~,ind]=min(abs(ang_1-90));
x_1=x_1(ind);
y_1=y_1(ind);
% Corte con la curva del circuito
% (yi+tan(theta-pi/2)*(x-xi))^2 = R^2-(x-sign(xi)*L/2)^2
% yi^2+tan(theta-pi/2)^2*(x^2+xi^2-2*xi*x)+2*tan(theta-pi/2)*(x-xi)*yi = R^2-x^2-L^2/4+2*sign(xi)*L/2*x
% x = roots([tan(theta-pi/2)^2+1  -2*(xi*tan(theta-pi/2)^2+sign(xi)*L/2-tan(theta-pi/2)*yi)   yi^2+tan(theta-pi/2)^2*xi^2-R^2+L^2/4-2*tan(theta-pi/2)*xi*yi])
if abs(x_1)<=L/2
    xct=x_1;
    yct=y_1;
else
    x_2 = roots([tan(theta-pi/2)^2+1 ...
        -2*(xit*tan(theta-pi/2)^2+sign(xit)*L/2-tan(theta-pi/2)*yit) ...
        yit^2+tan(theta-pi/2)^2*xit^2-R^2+L^2/4-2*tan(theta-pi/2)*xit*yit]);
        [~,ind]=min(abs(x_2-xit));
    xct=x_2(ind);
    aux=sqrt(abs(R^2-(xct-sign(xit)*L/2)^2));
    y_2=[aux ; -aux];
    V1=[(xct-xit)+1j*(y_2(1)-yit) ; (xct-xit)+1j*(y_2(2)-yit)];
    V2=[d_sens/2*cos(theta)+1j*d_sens/2*sin(theta); d_sens/2*cos(theta)+1j*d_sens/2*sin(theta)];
    ang_2=angle(V2./V1)*180/pi;
    [~,ind]=min(abs(ang_2-90));
    yct=y_2(ind);
end
d2=norm([xct-xit ; yct-yit]);

%% Angulo con respecto al circuito
theta_circ=atan2(d1-d2,d_sens);

%% Distancia en m
d=(d1+d2)/2/cosd(theta_circ);
d1=d1;
d2=d2;

% Existencia de rampa
rampa=0;
if abs(xi)<=Lr/2 
   % El coche está en la rampa
   if yi<0
       % Rampa ascendente
       rampa=1;
   else
       % Rampa descendente
       rampa=-1;
   end
end
% Determinacion del estado
if abs(xi)<=L/2 
   % El coche está en el tramo recto
   if yi<0
       % Subida
       estado=est_ant+(rem(est_ant,4)==1);
   else
       % Bajada
       estado=est_ant+(rem(est_ant,4)==3);
   end
elseif xi>L/2
    % El coche está en la curva superior
       estado=est_ant+(rem(est_ant,4)==2);
else
    % El coche está en la curva inferior
    estado=est_ant+(rem(est_ant,4)==0);
end

== matlab function TEST_LIDAR/CONTROL/LOCAL TARGETS/OPL TARGETS/VOLTAGE PULSE GENERATION ==
  data: CONTROL input Bus: CONTROL_Bus; MOTOR_VOLT_TARGET output
function MOTOR_VOLT_TARGET = PULSE_VOLT_GEN(CONTROL)
    
persistent TIMER initialize
if isempty(initialize)
    TIMER = 0;
    initialize = 1;
end

% SAMPLING TIME
SAMPLING_TIME = CONTROL.PARAM.SAMPLING_TIME; % s

%% OPERATION MODE
% / 0. BOOTING   / 1. SENSOR CALIBRATION / 2. READY
% / 3. OPEN LOOP / 4. ATTITUDE / 5. VELOCITY / 6. NAVIGATION / 
% / 7. WALL FOLLOWER / 8. WALL-FOLLOWER COMPETITION / 
% / 9. NAVIGATION COMPETITION / 10. STOP
CURRENT_STATUS = CONTROL.STATE.CURRENT_STATUS_SYS;
PREVIOUS_STATUS = CONTROL.STATE.PREVIOUS_STATUS;

if (CURRENT_STATUS == 3)&&(PREVIOUS_STATUS == 3)   
    if TIMER > 6
        MOTOR_VOLT_TARGET = 0;
    elseif TIMER < 5
        MOTOR_VOLT_TARGET = 0;
        TIMER = TIMER + SAMPLING_TIME;
    else % 5 <= TIMER <= 6
        MOTOR_VOLT_TARGET = 4;
        TIMER = TIMER + SAMPLING_TIME;
    end
else
    MOTOR_VOLT_TARGET = 0;
    TIMER = 0;
end

== matlab function TEST_LIDAR/HARDWARE/COMMUNICATIONS/UART_MUX/MATLAB Function ==
  settings: updateMethod=DISCRETE  sampleTime=SAMPLING_TIME
  data: A output; B output; INH output; RCRX output; BL output
function [A,B,INH,RCRX,BL] = UART_MULTIPLEXER()

% Counter initialization
persistent initialize ii

if isempty(initialize)
    count = 0;
    initialize = true;
end

INH = false;
% Mux channel selection
switch count
    case 0
        A = false;
        B = false;
        BL = true;
        RCRX = false;
    case 1
        A = true;
        B = false;
        BL = false;
        RCRX = true;
    otherwise
        INH = true;
        A = false;
        B = false;
        BL = false;
        RCRX = false;
end
count = count + 1;
if count > 1 
    count = 0;
end
